simulink library "ovenLib"  (R2016a)
settings: Solver=ode45  StartTime=0.0  StopTime=10.0  RelTol=1e-3
undefined symbols (not defined in the file): des, N
libraries: fl_lib x33, simulink x18, nesl_utility x11, PJPhysLib_lib x3
(part 1 of 2)
settings Model: Creator=peter  LastModifiedBy=peter
settings DataIOCC: LimitDataPoints=on  SaveFormat=Array
settings HardwareCC: ProdBitPerPointer=32  ProdLargestAtomicFloat=None  ProdIntDivRoundTo=Undefined  ProdEndianess=Unspecified  ProdWordSize=32  ProdHWDeviceType=32-bit Generic
settings ModelReferenceCC: PropagateSignalLabelsOutOfModel=off
settings ConfigComp: CovModelRefEnable=Off

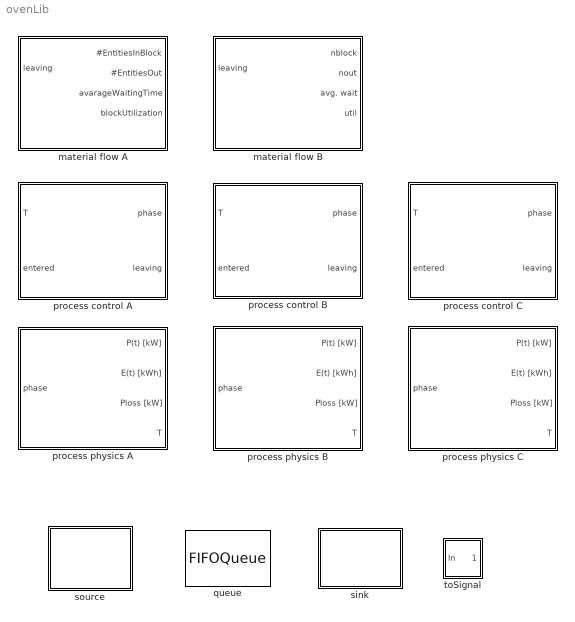
== system ovenLib ==
  material flow A : Subsystem  mask{N=6}
      mask prompts: N "oven capacity"
      mask Display:
      | text(0.1, 0.55, '\fontsize{24} MF (A)', 'texmode', 'on')
      | port_label('input', 1, 'leaving')
      | port_label('output', 2, 'nOut')
      | port_label('output', 1, 'nBlock')
      | port_label('output', 3, 'avg. wait')
      | port_label('output', 4, 'util.')
  material flow B : Subsystem  mask{N=N}
      mask prompts: N "oven capacity"
      mask Display:
      | text(0.1, 0.55, '\fontsize{24} MF (B)', 'texmode', 'on')
      | port_label('input', 1, 'leaving')
      | port_label('output', 2, 'nOut')
      | port_label('output', 1, 'nBlock')
      | port_label('output', 3, 'avg. wait')
      | port_label('output', 4, 'util.')
  process control A : Subsystem  mask{tH=70, Tset=800, N=6}
      mask prompts: tH "heating time [min]"; Tset "heating temperature [°C]"; N "oven capacity"
      mask Display:
      | disp('\fontsize{24} PC (A)', 'texmode', 'on')
      | port_label('input', 1, 'T')
      | port_label('input', 2, 'entered')
      | port_label('output', 1, 'phase')
      | port_label('output', 2, 'leaving')
  process control B : Subsystem  mask{HeatProgram=[40 400; 30 800], N=6}
      mask prompts: HeatProgram "heating program"; N "oven capacity"
      mask Display:
      | disp('\fontsize{24} PC (B)', 'texmode', 'on')
      | port_label('input', 1, 'T')
      | port_label('input', 2, 'entered')
      | port_label('output', 1, 'phase')
      | port_label('output', 2, 'leaving')
  process control C : Subsystem  mask{T0C=0, Tcool=30, N=6, HeatProgram=[0 20; 30 400;70 400;110 800;140 800]}
      mask prompts: T0C "0 °C in K"; Tcool "cooling temperature [°C]"; N "oven capacity"; HeatProgram "heating program"
      mask init:
      | T0C = 273.15;
      mask Display:
      | disp('\fontsize{24} PC (C)', 'texmode', 'on')
      | port_label('input', 1, 'T')
      | port_label('input', 2, 'entered')
      | port_label('output', 1, 'phase')
      | port_label('output', 2, 'leaving')
  process physics A : Subsystem  mask{Te=20, T_o=20, m_o=70, PH=8000, cp_o=1000, k_A=6.4, P0=2000}
      mask prompts: Te "environment temperature [°C]"; T_o "initial oven temperature [°C]"; m_o "oven mass [kg]"; PH "heating power [W]"; cp_o "oven specific heat capacity [J/(kg*K)]"; k_A "heat transfer coefficient * area [W/K]"; P0 "basic oven load [W]"
      mask init:
      | T0C = 273.15;
      | sigma = 5.67e-8;
      mask Display:
      | text(0.2, 0.55, '\fontsize{24} PP (A)', 'texmode', 'on')
      | port_label('input', 1, 'phase')
      | port_label('output', 1, 'P(t)')
      | port_label('output', 2, 'E(t)')
      | port_label('output', 3, 'Ploss(t)')
      | port_label('output', 4, 'T')
  process physics B : Subsystem  mask{T0C=0, sigma=0, Tu=20, T_o=20, m_o=70, PH=8000, cp_o=1000, etaO=0.95, alpha=28, epsilon=0.22, k_A=6.4, A_t=0.2, Pgrund=2000, m_w=1.4, cp_w=480, A_w_k=0.02, A_w_s=0.02, T_w=20}
      mask prompts: T0C "0°C in K"; sigma "Stefan Boltzmann constant"; Tu "environment temperature [°C]"; T_o "initial oven temperature [°C]"; m_o "oven mass [kg]"; PH "heating power [W]"; cp_o "oven specific heat capacity [J/(kg*K)]"; etaO "oven efficiency"; alpha "heat transfer coefficient [W/(m^2*K)]"; epsilon "emissivity"; k_A "heat transfer coefficient * area [W/K]"; A_t "area of oven door [m^2]"; Pgrund "basic oven load [W]"; m_w "work piece mass [kg]"; cp_w "work piece specific heat capacity [J/(kg*K)]"; A_w_k "work piece convective area [m^2]"; A_w_s "work piece radiation area [m^2]"; T_w "initial work piece temperature [°C]"
      mask init:
      | T0C = 273.15;
      | sigma = 5.67e-8;
      mask Display:
      | text(0.2, 0.55, '\fontsize{24} PP (B)', 'texmode', 'on')
      | port_label('input', 1, 'phase')
      | port_label('output', 1, 'P(t)')
      | port_label('output', 2, 'E(t)')
      | port_label('output', 3, 'Ploss(t)')
      | port_label('output', 4, 'T')
  process physics C : Subsystem  mask{T0C=0, sigma=0, Tu=20, T_o=20, m_o=70, PH=8000, cp_o=1000, etaO=0.95, alpha=28, epsilon=0.22, k_A=6.4, A_t=0.2, Pgrund=2000, m_w=1.4, cp_w=480, A_w_k=0.02, A_w_s=0.02, T_w=20}
      mask prompts: T0C "0°C in K"; sigma "Stefan Boltzmann constant"; Tu "environment temperature [°C]"; T_o "initial oven temperature [°C]"; m_o "oven mass [kg]"; PH "heating power [W]"; cp_o "oven specific heat capacity [J/(kg*K)]"; etaO "oven efficiency"; alpha "heat transfer coefficient [W/(m^2*K)]"; epsilon "emissivity"; k_A "heat transfer coefficient * area [W/K]"; A_t "area of oven door [m^2]"; Pgrund "basic oven load [W]"; m_w "work piece mass [kg]"; cp_w "work piece specific heat capacity [J/(kg*K)]"; A_w_k "work piece convective area [m^2]"; A_w_s "work piece radiation area [m^2]"; T_w "initial work piece temperature [°C]"
      mask init:
      | T0C = 273.15;
      | sigma = 5.67e-8;
      mask Display:
      | text(0.2, 0.55, '\fontsize{24} PP (C)', 'texmode', 'on')
      | port_label('input', 1, 'phase')
      | port_label('output', 1, 'P(t)')
      | port_label('output', 2, 'E(t)')
      | port_label('output', 3, 'Ploss(t)')
      | port_label('output', 4, 'T')
  queue : FIFOQueue  Capacity=inf
  sink : Subsystem  mask{nParts=25}
      mask prompts: nParts "Anzahl der bearbeiteten Werkstuecke"
  source : Subsystem  mask{nParts=25, period=0.1, parts=|, htz=100Cr6}
      mask parts=|
      | [-110 -110    0    0 -110    0    0    0    0    0    0    0    0    0    0    0    0    0    0    0
      |    0   60   60    0    0    0    0    0    0    0    0    0    0    0    0    0    0    0    0    0
      |    0    0    0    0    0    0    0    0    0    0    0    0    0    0    0    0    0    0    0    0
      |    0    0    0    0    0    0    0    0    0    0    0    0    0    0    0    0    0    0    0    0
      | ]
      mask prompts: nParts "Anzahl der zu generierende Werkstuecke"; period "Transferzeit in [s]"; parts "Rohteilgeometrie"; htz "Werkstoff"
      mask TypeOptions htz: 100Cr6 | 42CrMo4
  toSignal : Subsystem

== system ovenLib/material flow A ==
  leaving : Inport
  N-Server : NServer  NumberOfServers=N  ServiceTime=0  StatNumberDeparted=on  StatNumberInBlock=on  StatAverageWait=on  StatUtilization=on
      settings: OutputPortMap=o0,o1,o4,o5
  Release Gate : ReleaseGate  OpenGateUpon=Function call from port fcn
  IN : PMIOPort  Port=1  Side=Left
  OUT : PMIOPort  Port=2  Side=Right
  #EntitiesInBlock : Outport
  #EntitiesOut : Outport  Port=2
  avarageWaitingTime : Outport  Port=3
  blockUtilization : Outport  Port=4
  wires:
  leaving/1 -> Release Gate/1
  N-Server/3 -> avarageWaitingTime/1
  N-Server/1 -> #EntitiesOut/1
  N-Server/2 -> #EntitiesInBlock/1
  N-Server/4 -> blockUtilization/1
  connections:
  IN/RConn1 -- N-Server/LConn1
  N-Server/RConn1 -- Release Gate/LConn1
  Release Gate/RConn1 -- OUT/RConn1

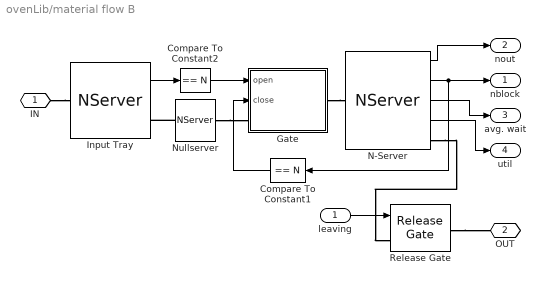
== system ovenLib/material flow B ==
  leaving : Inport
  Compare To Constant1 : simulink/Logic and Bit Operations/Compare To Constant  relop===  const=N  OutDataTypeStr=boolean
  Compare To Constant2 : simulink/Logic and Bit Operations/Compare To Constant  relop===  const=N  OutDataTypeStr=boolean
  Gate : Subsystem  mask(Gate){}
      mask help:
      | Gate for Entities that can be opened or closed via rising trigger inputs.
      | It is  initially open.
  Input Tray : NServer  NumberOfServers=N  ServiceTime=0  StatNumberInBlock=on
      settings: OutputPortMap=o1
  N-Server : NServer  NumberOfServers=N  ServiceTime=0  StatNumberDeparted=on  StatNumberInBlock=on  StatAverageWait=on  StatUtilization=on
      settings: OutputPortMap=o0,o1,o4,o5
  Nullserver : NServer  NumberOfServers=1  ServiceTime=0
  Release Gate : ReleaseGate  OpenGateUpon=Function call from port fcn
  IN : PMIOPort  Port=1  Side=Left
  OUT : PMIOPort  Port=2  Side=Right
  nblock : Outport
  nout : Outport  Port=2
  avg. wait : Outport  Port=3
  util : Outport  Port=4
  wires:
  Input Tray/1 -> Compare To Constant2/1
  Compare To Constant2/1 -> Gate/1(open)
  leaving/1 -> Release Gate/1
  Compare To Constant1/1 -> Gate/2(close)
  N-Server/1 -> nout/1
  N-Server/3 -> avg. wait/1
  N-Server/2 -> Compare To Constant1/1, nblock/1
  N-Server/4 -> util/1
  connections:
  Nullserver/RConn1 -- Gate/LConn1
  Nullserver/LConn1 -- Input Tray/RConn1
  Release Gate/RConn1 -- OUT/RConn1
  Gate/RConn1 -- N-Server/LConn1
  IN/RConn1 -- Input Tray/LConn1
  N-Server/RConn1 -- Release Gate/LConn1

== system ovenLib/process control A ==
  T : Inport
  entered : Inport  Port=2
  Constant1 : Constant  Value=0
  Event to Timed Signal1 : EventToTimedSignal
  MinMax : MinMax  Function=max  Inputs=5
  create control entity : Subsystem
  destroy control entity : Subsystem
  gate control : Subsystem  TreatAsAtomicUnit=on
  phase 1 load : Subsystem  mask{ts=5}
      mask prompts: ts "Service Time [min]"
  phase 2 heatUp : Subsystem
  phase 3 hold : Subsystem
  phase 4 unload : Subsystem  mask{ts=5}
      mask prompts: ts "Service Time [min]"
  phase : Outport
  leaving : Outport  Port=2
  wires:
  T/1 -> phase 2 heatUp/1(T)
  phase 1 load/1(Phase) -> MinMax/2
  phase 2 heatUp/1(Phase) -> MinMax/3
  phase 3 hold/1(Phase) -> MinMax/4
  Constant1/1 -> MinMax/1
  MinMax/1 -> Event to Timed Signal1/1
  phase 4 unload/1(Phase) -> MinMax/5
  gate control/1(fN) -> leaving/1
  Event to Timed Signal1/1 -> phase/1
  entered/1 -> create control entity/1(#n)
  destroy control entity/1(trigger) -> gate control/Trigger
  connections:
  phase 3 hold/LConn1 -- phase 2 heatUp/RConn1
  phase 3 hold/RConn1 -- phase 4 unload/LConn1
  phase 1 load/RConn1 -- phase 2 heatUp/LConn1
  create control entity/RConn1 -- phase 1 load/LConn1
  destroy control entity/LConn1 -- phase 4 unload/RConn1

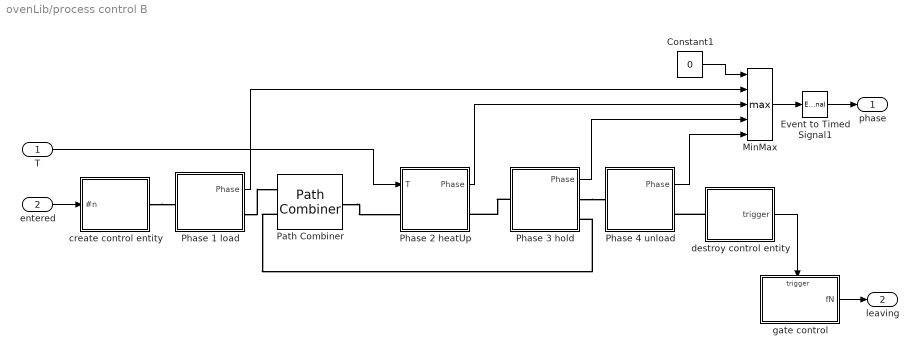
== system ovenLib/process control B ==
  T : Inport
  entered : Inport  Port=2
  Constant1 : Constant  Value=0
  Event to Timed Signal1 : EventToTimedSignal
  MinMax : MinMax  Function=max  Inputs=5
  Path Combiner : PathCombiner  NumberInputPorts=2
  Phase 1 load : Subsystem  mask{ts=5}
      mask prompts: ts "Service Time [min]"
  Phase 2 heatUp : Subsystem
  Phase 3 hold : Subsystem
  Phase 4 unload : Subsystem  mask{ts=5}
      mask prompts: ts "Service Time [min]"
  create control entity : Subsystem
  destroy control entity : Subsystem
  gate control : Subsystem  TreatAsAtomicUnit=on
  phase : Outport
  leaving : Outport  Port=2
  wires:
  destroy control entity/1(trigger) -> gate control/Trigger
  entered/1 -> create control entity/1(#n)
  Event to Timed Signal1/1 -> phase/1
  gate control/1(fN) -> leaving/1
  T/1 -> Phase 2 heatUp/1(T)
  Phase 4 unload/1(Phase) -> MinMax/5
  MinMax/1 -> Event to Timed Signal1/1
  Constant1/1 -> MinMax/1
  Phase 3 hold/1(Phase) -> MinMax/4
  Phase 2 heatUp/1(Phase) -> MinMax/3
  Phase 1 load/1(Phase) -> MinMax/2
  connections:
  destroy control entity/LConn1 -- Phase 4 unload/RConn1
  create control entity/RConn1 -- Phase 1 load/LConn1
  Path Combiner/RConn1 -- Phase 2 heatUp/LConn1
  Path Combiner/LConn2 -- Phase 3 hold/RConn2
  Phase 3 hold/RConn1 -- Phase 4 unload/LConn1
  Phase 1 load/RConn1 -- Path Combiner/LConn1
  Phase 3 hold/LConn1 -- Phase 2 heatUp/RConn1

== system ovenLib/process control C ==
  T : Inport
  entered : Inport  Port=2
  Constant16 : Constant  Value=N
  Constant17 : Constant  Value=HeatProgram
  DEVS : Stateflow chart  TreatAsAtomicUnit=on
  Event to Timed Signal1 : EventToTimedSignal
  Event to Timed Signal2 : EventToTimedSignal
  Mux : Mux
  Signal-Based Function-Call Generator : SignalBasedFunctionCallGenerator
      settings: InputPortMap=u1
  checkTemperature : Subsystem
  schedTEvent : Subsystem
  phase : Outport
  leaving : Outport  Port=2
  wires:
  entered/1 -> Signal-Based Function-Call Generator/1
  Event to Timed Signal2/1 -> phase/1, checkTemperature/1(phase)
  Event to Timed Signal1/1 -> checkTemperature/2(Tset)
  checkTemperature/2(coolDownReady) -> Mux/4
  checkTemperature/1(heatUpReady) -> Mux/3
  schedTEvent/1(wakeUp) -> Mux/2
  Signal-Based Function-Call Generator/1 -> Mux/1
  DEVS/2(Tset) -> Event to Timed Signal1/1
  Constant17/1 -> DEVS/2(HeatP)
  Constant16/1 -> DEVS/1(max_capa)
  DEVS/3(phase) -> Event to Timed Signal2/1
  DEVS/4(newSigma()) -> schedTEvent/1(newSigma)
  DEVS/1(sigma) -> schedTEvent/2(sigma)
  DEVS/5(openGate()) -> leaving/1
  Mux/1 -> DEVS/Trigger
  T/1 -> checkTemperature/3(T)

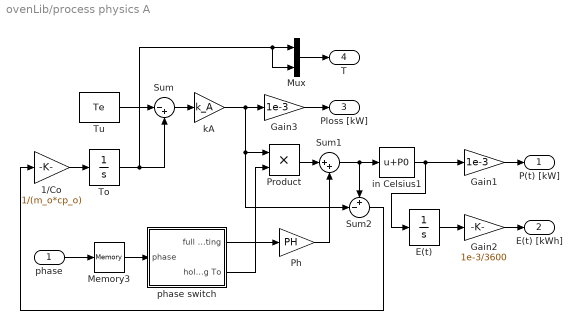
== system ovenLib/process physics A ==
  phase : Inport
  1/Co : Gain  Gain=1/(m_o*cp_o)
  E(t) : Integrator
  Gain1 : Gain  Gain=1e-3
  Gain2 : Gain  Gain=1e-3/3600
  Gain3 : Gain  Gain=1e-3
  Memory3 : Memory  InheritSampleTime=on
  Mux : Mux  Inputs=2
  Ph : Gain  Gain=PH
  Product : Product
  Sum : Sum  Inputs=|-+
  Sum1 : Sum  Inputs=|++
  Sum2 : Sum  Inputs=+-|
  To : Integrator  InitialCondition=T_o
  Tu : Constant  Value=Te
  in Celsius1 : Bias  Bias=P0
  kA : Gain  Gain=k_A
  phase switch : Subsystem
  P(t) [kW] : Outport
  E(t) [kWh] : Outport  Port=2
  Ploss [kW] : Outport  Port=3
  T : Outport  Port=4
  wires:
  Gain2/1 -> E(t) [kWh]/1
  E(t)/1 -> Gain2/1
  in Celsius1/1 -> E(t)/1, Gain1/1
  Sum/1 -> kA/1
  Gain3/1 -> Ploss [kW]/1
  Gain1/1 -> P(t) [kW]/1
  Memory3/1 -> phase switch/1(phase)
  phase/1 -> Memory3/1
  Sum2/1 -> 1/Co/1
  1/Co/1 -> To/1
  Sum1/1 -> in Celsius1/1, Sum2/1
  Product/1 -> Sum1/1
  Ph/1 -> Sum1/2
  phase switch/1(full heating) -> Ph/1
  phase switch/2(holding To) -> Product/2
  kA/1 -> Sum2/2, Product/1, Gain3/1
  Tu/1 -> Sum/1
  To/1 -> Sum/2, Mux/1, Mux/2
  Mux/1 -> T/1

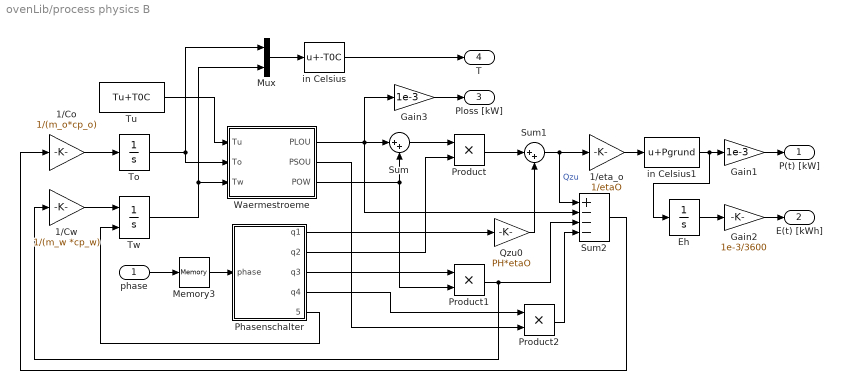
== system ovenLib/process physics B ==
  phase : Inport
  1/Co : Gain  Gain=1/(m_o*cp_o)
  1/Cw : Gain  Gain=1/(m_w *cp_w)
  1/eta_o : Gain  Gain=1/etaO
  Eh : Integrator
  Gain1 : Gain  Gain=1e-3
  Gain2 : Gain  Gain=1e-3/3600
  Gain3 : Gain  Gain=1e-3
  Memory3 : Memory  InheritSampleTime=on
  Mux : Mux  Inputs=2
  Phasenschalter : Subsystem
  Product : Product
  Product1 : Product
  Product2 : Product
  Qzu0 : Gain  Gain=PH*etaO
  Sum : Sum  Inputs=|++
  Sum1 : Sum  Inputs=|++
  Sum2 : Sum  Inputs=+---
  To : Integrator  InitialCondition=T_w + T0C
  Tu : Constant  Value=Tu+T0C
  Tw : Integrator  ExternalReset=rising  InitialCondition=T_w + T0C
  Waermestroeme : Subsystem
  in Celsius : Bias  Bias=-T0C
  in Celsius1 : Bias  Bias=Pgrund
  P(t) [kW] : Outport
  E(t) [kWh] : Outport  Port=2
  Ploss [kW] : Outport  Port=3
  T : Outport  Port=4
  wires:
  Gain2/1 -> E(t) [kWh]/1
  Eh/1 -> Gain2/1
  Gain3/1 -> Ploss [kW]/1
  Gain1/1 -> P(t) [kW]/1
  Memory3/1 -> Phasenschalter/1(phase)
  phase/1 -> Memory3/1
  To/1 -> Mux/1, Waermestroeme/2(To)
  Phasenschalter/5(restartTw) -> Tw/2
  Phasenschalter/4(q4) -> Product2/1
  in Celsius1/1 -> Gain1/1, Eh/1
  1/eta_o/1 -> in Celsius1/1
  Sum2/1 -> 1/Co/1
  Product2/1 -> Sum2/4
  Waermestroeme/2(PSOU) -> Product2/2
  Product1/1 -> Sum2/3, 1/Cw/1
  Phasenschalter/3(q3) -> Product1/1
  1/Cw/1 -> Tw/1
  1/Co/1 -> To/1
  Sum1/1 -> Sum2/1, 1/eta_o/1  "Qzu"
  Product/1 -> Sum1/1
  Qzu0/1 -> Sum1/2
  Phasenschalter/1(q1) -> Qzu0/1
  Phasenschalter/2(q2) -> Product/2
  Sum/1 -> Product/1
  Waermestroeme/3(POW) -> Sum/2, Product1/2
  Waermestroeme/1(PLOU) -> Gain3/1, Sum2/2, Sum/1
  Tu/1 -> Waermestroeme/1(Tu)
  in Celsius/1 -> T/1
  Mux/1 -> in Celsius/1
  Tw/1 -> Waermestroeme/3(Tw), Mux/2

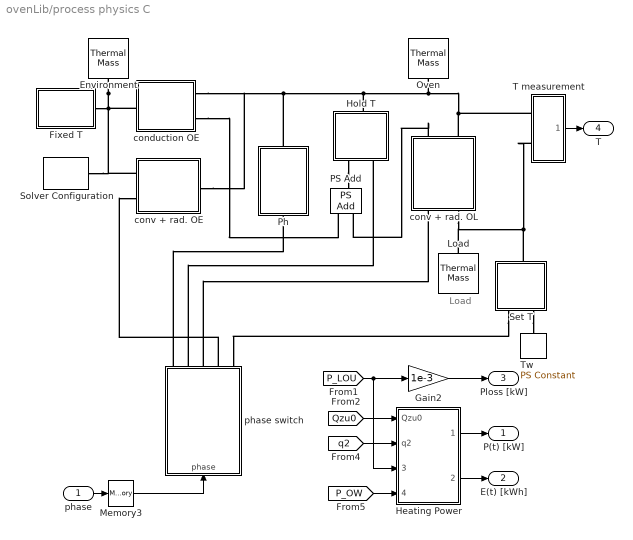
== system ovenLib/process physics C ==
  note: Load
  phase : Inport
  Environment : fl_lib/Thermal/Thermal Elements/Thermal Mass  mass=1000 kg  sp_heat=2000 J/kg/K  T_specify=on  T_priority=High  T=360 K  Q_specify=off  Q_priority=High  Q=0 J/s
  Fixed T : Subsystem
  Gain2 : Gain  Gain=1e-3
  Heating Power : Subsystem
  Hold T : Subsystem
  Load : fl_lib/Thermal/Thermal Elements/Thermal Mass  mass=m_w kg  sp_heat=cp_w J/kg/K  T_specify=on  T_priority=High  T=T_w K  Q_specify=off  Q_priority=High  Q=0 J/s
  Memory3 : Memory  InheritSampleTime=on
  Oven : fl_lib/Thermal/Thermal Elements/Thermal Mass  mass=m_o kg  sp_heat=cp_o J/kg/K  T_specify=on  T_priority=High  T=T_o K  Q_specify=off  Q_priority=High  Q=0 J/s
  PS Add : fl_lib/Physical Signals/Functions/PS Add
  Ph : Subsystem
  Set T : Subsystem
  Solver Configuration : nesl_utility/Solver Configuration  PhysicalDomain=network_engine_domain  SubClassName=solver  LeftPortType=input  RightPortType=generic  Accelerate=off  Tones=[]  Harmonics=[]  SimulateNoise=off  Profile=off  UseLocalSampling=off  EnableSwitchedLinearOptims=on  FrequencyDomain=off  UseCCode=off  RelTol=0.001  AbsTol=1e-06  MinStep=1e-09  ToWorkspace=off  RevertToSquareIcSolve=off  NumHomotopyIterations=100  PhasorMode=off  PhasorModeNumHarmonics=1  OverrideAbsTol=off  DoDC=off  ResidualTolerance=1e-09  UseLocalSolver=off  LocalSolverChoice=NE_BACKWARD_EULER_ADVANCER  LocalSolverSampleTime=0.001  DoFixedCost=off  MaxNonlinIter=3  MaxModeIter=2  LinearAlgebra=Sparse  DelaysMemoryBudget=1024  AutomaticFiltering=on  FilteringTimeConstant=0.001
  T measurement : Subsystem
      mask Display: image('thermometer.png')
  Tw : fl_lib/Physical Signals/Sources/PS Constant  constant=T_w + T0C
  conduction OE : Subsystem
  conv + rad. OL : Subsystem
  conv + rad. OE : Subsystem
  phase switch : Subsystem
  P(t) [kW] : Outport
  E(t) [kWh] : Outport  Port=2
  Ploss [kW] : Outport  Port=3
  T : Outport  Port=4
  wires:
  Heating Power/2(E(t) [kWh]) -> E(t) [kWh]/1
  Gain2/1 -> Ploss [kW]/1
  Heating Power/1(P(t) [kW]) -> P(t) [kW]/1
  [Qzu0] -> Heating Power/1(Qzu0)
  [q2] -> Heating Power/2(q2)
  [P_LOU] -> Heating Power/3(P_LOU), Gain2/1
  [P_OW] -> Heating Power/4(P_OW)
  phase/1 -> Memory3/1
  Memory3/1 -> phase switch/1(phase)
  T measurement/1(Out1) -> T/1
  connections:
  Environment/LConn1 -- conv + rad. OE/LConn1 -- Solver Configuration/RConn1 -- conduction OE/LConn1 -- Fixed T/RConn1
  Ph/RConn1 -- conv + rad. OE/RConn1 -- conduction OE/RConn1 -- Oven/LConn1 -- T measurement/LConn1 -- conv + rad. OL/RConn2 -- Hold T/RConn1
  Set T/RConn1 -- T measurement/LConn2 -- Load/LConn1 -- conv + rad. OL/LConn2
  Set T/LConn1 -- phase switch/RConn5
  Set T/LConn2 -- Tw/RConn1
  conduction OE/RConn2 -- PS Add/LConn2
  conv + rad. OL/RConn1 -- PS Add/LConn1
  phase switch/RConn1 -- Ph/LConn1
  Hold T/LConn1 -- PS Add/RConn1
  phase switch/RConn4 -- conv + rad. OE/LConn2
  phase switch/RConn3 -- conv + rad. OL/LConn1
  phase switch/RConn2 -- Hold T/LConn2

== system ovenLib/sink ==
  Constant : Constant  Value=nParts
  Entity Sink : EntitySink  StatNumberArrived=on
  Event to Timed Signal : EventToTimedSignal
  Relational Operator : RelationalOperator  Operator===  OutDataTypeStr=boolean
  Stop Simulation : Stop
  IN : PMIOPort  Port=1  Side=Left
  wires:
  Relational Operator/1 -> Event to Timed Signal/1
  Event to Timed Signal/1 -> Stop Simulation/1
  Constant/1 -> Relational Operator/1
  Entity Sink/1 -> Relational Operator/2
  connections:
  IN/RConn1 -- Entity Sink/LConn1

== system ovenLib/source ==
  Attribute Function : Subsystem  LoadFcn=des.afb.attributefunction_support(gcb,'LoadFcn');  StartFcn=des.afb.attributefunction_support(gcb,'StartFcn');  mask(Attribute Function){OutputNamePrefix=out_}
      mask prompts: OutputNamePrefix "Prefix name"
      settings: CopyFcn=des.afb.attributefunction_support(gcb,'CopyFcn');  OpenFcn=des.afb.attributefunction_support(gcb,'OpenFcn');  ErrorFcn=des.afb.error_redirect
      mask Help: slhelp(gcbh)
      mask Display: image(des_iconLoad('attribFunction.jpg'),'center');
  Constant : Constant  Value=nParts
  Constant1 : Constant  Value=htz
  Constant2 : Constant  Value=parts
  Entity Departure Counter : EntityDepartureCounter  NumberDepartedAttributeName=part_no
  Entity Sink : EntitySink  AvailableForArrivals=off
  Output Switch : OutputSwitch  NumberOutputPorts=2  SwitchingCriterion=From attribute  AttributeName=port
  Set Attribute : SetAttribute  AttributeName=nr_wp  AttributeFrom=Signal port  EvaluatedAttributeValue={ []}
  Set Attribute1 : SetAttribute  AttributeName=htz|parts  AttributeFrom=Signal port|Signal port  AttributeValue=1|1  AttributeTreatAsVector=1|1  EvaluatedAttributeValue={ [];[]}
      settings: InputPortMap=u0,u1
  Single Server1 : SingleServer  ServiceTime=0
  Time-Based Entity Generator : TimeBasedEntityGenerator  Period=period
  OUT : PMIOPort  Port=1  Side=Right
  wires:
  Constant2/1 -> Set Attribute1/2
  Constant1/1 -> Set Attribute1/1
  Constant/1 -> Set Attribute/1
  connections:
  Time-Based Entity Generator/RConn1 -- Entity Departure Counter/LConn1
  Entity Departure Counter/RConn1 -- Set Attribute/LConn1
  Attribute Function/RConn1 -- Single Server1/LConn1
  Set Attribute/RConn1 -- Attribute Function/LConn1
  Output Switch/RConn1 -- Set Attribute1/LConn1
  Output Switch/RConn2 -- Entity Sink/LConn1
  Set Attribute1/RConn1 -- OUT/RConn1
  Single Server1/RConn1 -- Output Switch/LConn1

== system ovenLib/toSignal ==
  In : Inport
  toSIgnal : EventToTimedSignal
  Out : Outport
  wires:
  toSIgnal/1 -> Out/1
  In/1 -> toSIgnal/1

== system ovenLib/material flow B/Gate ==
  open : Inport
  close : Inport  Port=2
  Constant : Constant  Value=0
  Constant1 : Constant
  Enabled Gate1 : EnabledGate
  Signal Latch : SignalLatch  WriteMemoryUpon=Trigger from port wtr  ReadMemoryUpon=Trigger from port rtr  MemoryReadEdgeOption=Rising  ReportMemoryState=on  ReportMemoryUponRead=off
      settings: InputPortMap=u0,u1,u2
  Sum : Sum  Inputs=+-|
  IN : PMIOPort  Port=1  Side=Left
  OUT : PMIOPort  Port=2  Side=Right
  wires:
  Sum/1 -> Enabled Gate1/1
  Constant1/1 -> Sum/1
  Signal Latch/1 -> Sum/2
  open/1 -> Signal Latch/2
  close/1 -> Signal Latch/1
  Constant/1 -> Signal Latch/3
  connections:
  Enabled Gate1/LConn1 -- IN/RConn1
  OUT/RConn1 -- Enabled Gate1/RConn1

== system ovenLib/process control A/create control entity ==
  #n : Inport
  Compare To Constant : simulink/Logic and Bit Operations/Compare To Constant  relop===  const=N  OutDataTypeStr=boolean
  Event-Based Entity Generator : EventBasedEntityGenerator
  OUT : PMIOPort  Port=1  Side=Right
  wires:
  #n/1 -> Compare To Constant/1
  Compare To Constant/1 -> Event-Based Entity Generator/1
  connections:
  Event-Based Entity Generator/RConn1 -- OUT/RConn1

== system ovenLib/process control A/destroy control entity ==
  Entity Sink : EntitySink  StatNumberArrived=on
  Signal-Based Function-Call Generator : SignalBasedFunctionCallGenerator
      settings: InputPortMap=u1
  IN : PMIOPort  Port=1  Side=Left
  trigger : Outport
  wires:
  Signal-Based Function-Call Generator/1 -> trigger/1
  Entity Sink/1 -> Signal-Based Function-Call Generator/1
  connections:
  Entity Sink/LConn1 -- IN/RConn1

== system ovenLib/process control A/gate control ==
  Trigger : TriggerPort  TriggerType=function-call  VariantControl=Variant
  Function-Call Generator : simulink/Ports & Subsystems/Function-Call Generator  sample_time=-1  numberOfIterations=N
  fN : Outport
  wires:
  Function-Call Generator/1 -> fN/1

== system ovenLib/process control A/phase 1 load ==
  Server load : SingleServer  ServiceTime=60*ts  StatNumberInBlock=on
      settings: OutputPortMap=o1
  phase : Gain
  OUT : PMIOPort  Port=1  Side=Right
  IN : PMIOPort  Port=2  Side=Left
  Phase : Outport
  wires:
  Server load/1 -> phase/1
  phase/1 -> Phase/1
  connections:
  IN/RConn1 -- Server load/LConn1
  Server load/RConn1 -- OUT/RConn1

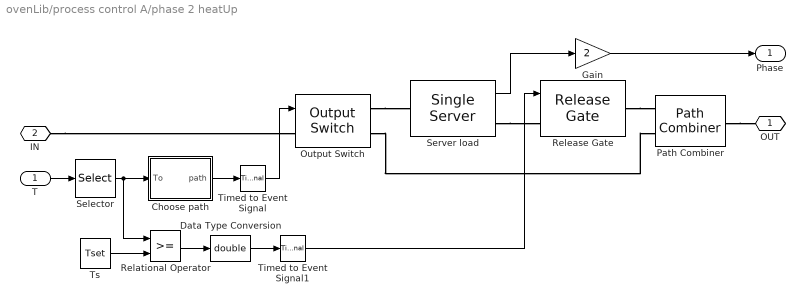
== system ovenLib/process control A/phase 2 heatUp ==
  T : Inport
  Choose path : Subsystem
  Data Type Conversion : DataTypeConversion  OutDataTypeStr=double
  Gain : Gain  Gain=2
  Output Switch : OutputSwitch  NumberOutputPorts=2  SwitchingCriterion=From signal port p  InitialConditionsOpt=on
  Path Combiner : PathCombiner  NumberInputPorts=2
  Relational Operator : RelationalOperator  OutDataTypeStr=boolean
  Release Gate : ReleaseGate
  Selector : Selector  InputPortWidth=2  IndexOptions=Index vector (dialog)  Indices=[1]  OutputSizes=1
  Server load : SingleServer  ServiceTime=0  StatNumberInBlock=on
      settings: OutputPortMap=o1
  Timed to Event Signal : TimedToEventSignal
  Timed to Event Signal1 : TimedToEventSignal
  Ts : Constant  Value=Tset
  OUT : PMIOPort  Port=1  Side=Right
  IN : PMIOPort  Port=2  Side=Left
  Phase : Outport
  wires:
  Timed to Event Signal/1 -> Output Switch/1
  Timed to Event Signal1/1 -> Release Gate/1
  Data Type Conversion/1 -> Timed to Event Signal1/1
  Relational Operator/1 -> Data Type Conversion/1
  Ts/1 -> Relational Operator/2
  Server load/1 -> Gain/1
  Gain/1 -> Phase/1
  T/1 -> Selector/1
  Choose path/1(path) -> Timed to Event Signal/1
  Selector/1 -> Choose path/1(To), Relational Operator/1
  connections:
  Server load/RConn1 -- Release Gate/LConn1
  IN/RConn1 -- Output Switch/LConn1
  Output Switch/RConn1 -- Server load/LConn1
  Release Gate/RConn1 -- Path Combiner/LConn1
  Path Combiner/RConn1 -- OUT/RConn1
  Output Switch/RConn2 -- Path Combiner/LConn2

== system ovenLib/process control A/phase 3 hold ==
  Gain : Gain  Gain=3
  Server load : SingleServer  ServiceTime=tH*60  StatNumberInBlock=on
      settings: OutputPortMap=o1
  IN : PMIOPort  Port=1  Side=Left
  OUT1 : PMIOPort  Port=2  Side=Right
  Phase : Outport
  wires:
  Gain/1 -> Phase/1
  Server load/1 -> Gain/1
  connections:
  Server load/LConn1 -- IN/RConn1
  Server load/RConn1 -- OUT1/RConn1

== system ovenLib/process control A/phase 4 unload ==
  Gain : Gain  Gain=4
  Server load : SingleServer  ServiceTime=60*ts  StatNumberInBlock=on
      settings: OutputPortMap=o1
  OUT : PMIOPort  Port=1  Side=Right
  IN : PMIOPort  Port=2  Side=Left
  Phase : Outport
  wires:
  Server load/1 -> Gain/1
  Gain/1 -> Phase/1
  connections:
  Server load/RConn1 -- OUT/RConn1
  IN/RConn1 -- Server load/LConn1

== system ovenLib/process control B/Phase 1 load ==
  Server load : SingleServer  ServiceTime=60*ts  StatNumberInBlock=on
      settings: OutputPortMap=o1
  Set HeatP number : SetAttribute  AttributeName=nextHeatPNo|HeatP  AttributeFrom=Dialog|Dialog  AttributeValue=1|HeatProgram  AttributeTreatAsVector=1|1  EvaluatedAttributeValue={ 1;HeatProgram}
  phase : Gain
  OUT : PMIOPort  Port=1  Side=Right
  IN : PMIOPort  Port=2  Side=Left
  Phase : Outport
  wires:
  phase/1 -> Phase/1
  Server load/1 -> phase/1
  connections:
  Set HeatP number/RConn1 -- OUT/RConn1
  IN/RConn1 -- Server load/LConn1
  Server load/RConn1 -- Set HeatP number/LConn1

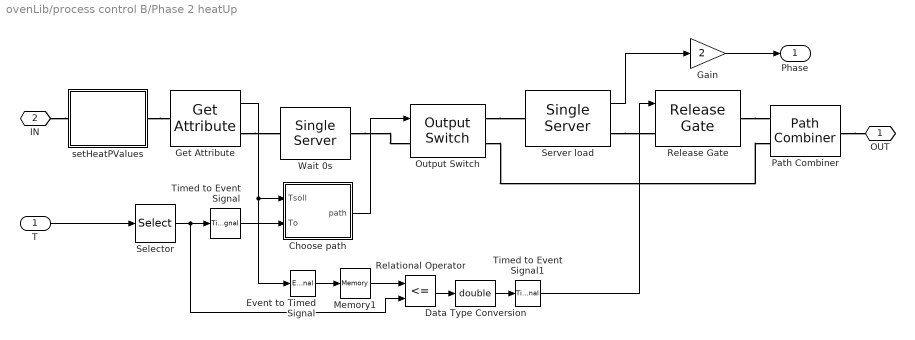
== system ovenLib/process control B/Phase 2 heatUp ==
  T : Inport
  Choose path : Subsystem  TreatAsAtomicUnit=on
  Data Type Conversion : DataTypeConversion  OutDataTypeStr=double
  Event to Timed Signal : EventToTimedSignal
  Gain : Gain  Gain=2
  Get Attribute : GetAttribute  AttributeName=HeatPTemp  EvaluatedDefaultAttributeValue={ []}
      settings: OutputPortMap=o1
  Memory1 : Memory
  Output Switch : OutputSwitch  NumberOutputPorts=2  SwitchingCriterion=From signal port p  InitialConditionsOpt=on
  Path Combiner : PathCombiner  NumberInputPorts=2
  Relational Operator : RelationalOperator  Operator=<=  OutDataTypeStr=boolean
  Release Gate : ReleaseGate
  Selector : Selector  InputPortWidth=2  IndexOptions=Index vector (dialog)  Indices=[1]  OutputSizes=1
  Server load : SingleServer  ServiceTime=0  StatNumberInBlock=on
      settings: OutputPortMap=o1
  Timed to Event Signal : TimedToEventSignal
  Timed to Event Signal1 : TimedToEventSignal
  Wait 0s : SingleServer  ServiceTime=0
  setHeatPValues : Subsystem  LoadFcn=des.afb.attributefunction_support(gcb,'LoadFcn');  StartFcn=des.afb.attributefunction_support(gcb,'StartFcn');  mask(Attribute Function){OutputNamePrefix=out_}
      mask prompts: OutputNamePrefix "Prefix name"
      settings: CopyFcn=des.afb.attributefunction_support(gcb,'CopyFcn');  OpenFcn=des.afb.attributefunction_support(gcb,'OpenFcn');  ErrorFcn=des.afb.error_redirect
      mask Help: slhelp(gcbh)
      mask Display: image(des_iconLoad('attribFunction.jpg'),'center');
  OUT : PMIOPort  Port=1  Side=Right
  IN : PMIOPort  Port=2  Side=Left
  Phase : Outport
  wires:
  Timed to Event Signal/1 -> Choose path/2(To)
  Timed to Event Signal1/1 -> Release Gate/1
  Data Type Conversion/1 -> Timed to Event Signal1/1
  Relational Operator/1 -> Data Type Conversion/1
  Event to Timed Signal/1 -> Memory1/1
  Memory1/1 -> Relational Operator/1
  T/1 -> Selector/1
  Selector/1 -> Relational Operator/2, Timed to Event Signal/1
  Choose path/1(path) -> Output Switch/1
  Get Attribute/1 -> Choose path/1(Tsoll), Event to Timed Signal/1
  Gain/1 -> Phase/1
  Server load/1 -> Gain/1
  connections:
  Get Attribute/RConn1 -- Wait 0s/LConn1
  Output Switch/RConn2 -- Path Combiner/LConn2
  Path Combiner/RConn1 -- OUT/RConn1
  Release Gate/RConn1 -- Path Combiner/LConn1
  Output Switch/RConn1 -- Server load/LConn1
  Wait 0s/RConn1 -- Output Switch/LConn1
  setHeatPValues/RConn1 -- Get Attribute/LConn1
  IN/RConn1 -- setHeatPValues/LConn1
  Server load/RConn1 -- Release Gate/LConn1

== system ovenLib/process control B/Phase 3 hold ==
  Gain : Gain  Gain=3
  Get Attribute : GetAttribute  AttributeName=HeatPTime  EvaluatedDefaultAttributeValue={ []}
      settings: OutputPortMap=o1
  Output Switch : OutputSwitch  NumberOutputPorts=2  SwitchingCriterion=From attribute  AttributeName=OutPort
  Server load : SingleServer  ServiceTimeFrom=Signal port t  ServiceTime=ts  StatNumberInBlock=on
      settings: OutputPortMap=o1
  Set Out Port : Subsystem  LoadFcn=des.afb.attributefunction_support(gcb,'LoadFcn');  StartFcn=des.afb.attributefunction_support(gcb,'StartFcn');  mask(Attribute Function){OutputNamePrefix=out_}
      mask prompts: OutputNamePrefix "Prefix name"
      settings: CopyFcn=des.afb.attributefunction_support(gcb,'CopyFcn');  OpenFcn=des.afb.attributefunction_support(gcb,'OpenFcn');  ErrorFcn=des.afb.error_redirect
      mask Help: slhelp(gcbh)
      mask Display: image(des_iconLoad('attribFunction.jpg'),'center');
  Sum : Sum  Inputs=|+++
  Wait 0s : SingleServer  ServiceTime=0  StatNumberInBlock=on
      settings: OutputPortMap=o1
  "Wait 0s " : SingleServer  ServiceTime=0  StatNumberInBlock=on
      settings: OutputPortMap=o1
  IN : PMIOPort  Port=1  Side=Left
  OUT1 : PMIOPort  Port=2  Side=Right
  OUT2 : PMIOPort  Port=3  Side=Right
  Phase : Outport
  wires:
  "Wait 0s "/1 -> Sum/3
  Server load/1 -> Sum/2
  Wait 0s/1 -> Sum/1
  Sum/1 -> Gain/1
  Get Attribute/1 -> Server load/1
  Gain/1 -> Phase/1
  connections:
  Server load/RConn1 -- Set Out Port/LConn1
  Output Switch/RConn1 -- OUT1/RConn1
  "Wait 0s "/RConn1 -- Output Switch/LConn1
  Output Switch/RConn2 -- OUT2/RConn1
  Set Out Port/RConn1 -- "Wait 0s "/LConn1
  Wait 0s/RConn1 -- Server load/LConn1
  Get Attribute/RConn1 -- Wait 0s/LConn1
  IN/RConn1 -- Get Attribute/LConn1

== system ovenLib/process control B/Phase 4 unload ==
  Gain : Gain  Gain=4
  Server load : SingleServer  ServiceTime=60*ts  StatNumberInBlock=on
      settings: OutputPortMap=o1
  OUT : PMIOPort  Port=1  Side=Right
  IN : PMIOPort  Port=2  Side=Left
  Phase : Outport
  wires:
  Gain/1 -> Phase/1
  Server load/1 -> Gain/1
  connections:
  IN/RConn1 -- Server load/LConn1
  Server load/RConn1 -- OUT/RConn1

== system ovenLib/process control B/create control entity ==
  #n : Inport
  Compare To Constant : simulink/Logic and Bit Operations/Compare To Constant  relop===  const=N  OutDataTypeStr=boolean
  Event-Based Entity Generator : EventBasedEntityGenerator
  Set Attribute : SetAttribute  AttributeName=BatchQuantity  AttributeValue=N  EvaluatedAttributeValue={ N}
  OUT : PMIOPort  Port=1  Side=Right
  wires:
  Compare To Constant/1 -> Event-Based Entity Generator/1
  #n/1 -> Compare To Constant/1
  connections:
  Set Attribute/RConn1 -- OUT/RConn1
  Event-Based Entity Generator/RConn1 -- Set Attribute/LConn1

== system ovenLib/process control B/destroy control entity ==
  Entity Sink : EntitySink  StatNumberArrived=on
  Signal-Based Function-Call Generator : SignalBasedFunctionCallGenerator
      settings: InputPortMap=u1
  IN : PMIOPort  Port=1  Side=Left
  trigger : Outport
  wires:
  Entity Sink/1 -> Signal-Based Function-Call Generator/1
  Signal-Based Function-Call Generator/1 -> trigger/1
  connections:
  Entity Sink/LConn1 -- IN/RConn1

== system ovenLib/process control B/gate control ==
  Trigger : TriggerPort  TriggerType=function-call  VariantControl=Variant
  Function-Call Generator : simulink/Ports & Subsystems/Function-Call Generator  sample_time=-1  numberOfIterations=N
  fN : Outport
  wires:
  Function-Call Generator/1 -> fN/1

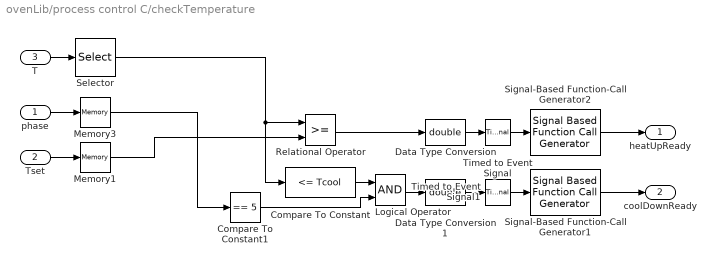
== system ovenLib/process control C/checkTemperature ==
  phase : Inport
  Tset : Inport  Port=2
  T : Inport  Port=3
  Compare To Constant : simulink/Logic and Bit Operations/Compare To Constant  relop=<=  const=Tcool  OutDataTypeStr=boolean
  Compare To Constant1 : simulink/Logic and Bit Operations/Compare To Constant  relop===  const=5  OutDataTypeStr=boolean
  Data Type Conversion : DataTypeConversion  OutDataTypeStr=double
  Data Type Conversion1 : DataTypeConversion  OutDataTypeStr=double
  Logical Operator : Logic  AllPortsSameDT=off  OutDataTypeStr=boolean
  Memory1 : Memory
  Memory3 : Memory  InheritSampleTime=on
  Relational Operator : RelationalOperator  OutDataTypeStr=boolean
  Selector : Selector  InputPortWidth=2  IndexOptions=Index vector (dialog)  Indices=[1]  OutputSizes=1
  Signal-Based Function-Call Generator1 : SignalBasedFunctionCallGenerator
      settings: InputPortMap=u1
  Signal-Based Function-Call Generator2 : SignalBasedFunctionCallGenerator
      settings: InputPortMap=u1
  Timed to Event Signal : TimedToEventSignal
  Timed to Event Signal1 : TimedToEventSignal
  heatUpReady : Outport
  coolDownReady : Outport  Port=2
  wires:
  Timed to Event Signal/1 -> Signal-Based Function-Call Generator2/1
  Signal-Based Function-Call Generator2/1 -> heatUpReady/1
  Data Type Conversion/1 -> Timed to Event Signal/1
  Relational Operator/1 -> Data Type Conversion/1
  Timed to Event Signal1/1 -> Signal-Based Function-Call Generator1/1
  Logical Operator/1 -> Data Type Conversion1/1
  Signal-Based Function-Call Generator1/1 -> coolDownReady/1
  phase/1 -> Memory3/1
  Compare To Constant/1 -> Logical Operator/1
  Compare To Constant1/1 -> Logical Operator/2
  Tset/1 -> Memory1/1
  Data Type Conversion1/1 -> Timed to Event Signal1/1
  Memory3/1 -> Compare To Constant1/1
  Memory1/1 -> Relational Operator/2
  T/1 -> Selector/1
  Selector/1 -> Compare To Constant/1, Relational Operator/1

== system ovenLib/process control C/schedTEvent ==
  newSigma : Inport
  sigma : Inport  Port=2
  Entity Departure Counter : EntityDepartureCounter
  Entity Departure Function-Call Generator1 : EntityDepartureFunctionCallGenerator
  Entity Sink2 : EntitySink
  Entity Sink3 : EntitySink
  Event-Based Entity Generator1 : EventBasedEntityGenerator  GenerateEntitiesUpon=Function call from port fcn
  Single Server1 : SingleServer  ServiceTimeFrom=Signal port t  PermitPreemption=on  SortingAttributeName=Count  SortingDirection=Descending
  wakeUp : Outport
  wires:
  Entity Departure Function-Call Generator1/1 -> wakeUp/1
  newSigma/1 -> Event-Based Entity Generator1/1
  sigma/1 -> Single Server1/1
  connections:
  Single Server1/RConn2 -- Entity Sink3/LConn1
  Entity Departure Counter/RConn1 -- Single Server1/LConn1
  Entity Departure Function-Call Generator1/RConn1 -- Entity Sink2/LConn1
  Entity Departure Counter/LConn1 -- Event-Based Entity Generator1/RConn1
  Single Server1/RConn1 -- Entity Departure Function-Call Generator1/LConn1

== system ovenLib/process physics A/phase switch ==
  phase : Inport
  Compare To Constant : simulink/Logic and Bit Operations/Compare To Constant  relop===  const=2  OutDataTypeStr=boolean
  Compare To Constant1 : simulink/Logic and Bit Operations/Compare To Constant  relop===  const=3  OutDataTypeStr=boolean
  Data Type Conversion : DataTypeConversion  OutDataTypeStr=double
  Data Type Conversion1 : DataTypeConversion  OutDataTypeStr=double
  full heating : Outport
  holding To : Outport  Port=2
  wires:
  Data Type Conversion1/1 -> holding To/1
  Compare To Constant1/1 -> Data Type Conversion1/1
  Data Type Conversion/1 -> full heating/1
  Compare To Constant/1 -> Data Type Conversion/1
  phase/1 -> Compare To Constant/1, Compare To Constant1/1

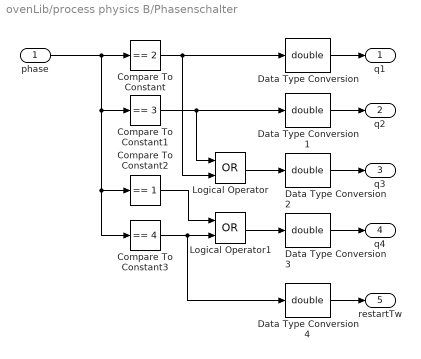
== system ovenLib/process physics B/Phasenschalter ==
  phase : Inport
  Compare To Constant : simulink/Logic and Bit Operations/Compare To Constant  relop===  const=2  OutDataTypeStr=boolean
  Compare To Constant1 : simulink/Logic and Bit Operations/Compare To Constant  relop===  const=3  OutDataTypeStr=boolean
  Compare To Constant2 : simulink/Logic and Bit Operations/Compare To Constant  relop===  const=1  OutDataTypeStr=boolean
  Compare To Constant3 : simulink/Logic and Bit Operations/Compare To Constant  relop===  const=4  OutDataTypeStr=boolean
  Data Type Conversion{,1..4} (5 alike) : DataTypeConversion  OutDataTypeStr=double
  Logical Operator : Logic  Operator=OR  AllPortsSameDT=off  OutDataTypeStr=boolean
  Logical Operator1 : Logic  Operator=OR  AllPortsSameDT=off  OutDataTypeStr=boolean
  q1 : Outport
  q2 : Outport  Port=2
  q3 : Outport  Port=3
  q4 : Outport  Port=4
  restartTw : Outport  Port=5
  wires:
  Data Type Conversion4/1 -> restartTw/1
  Compare To Constant2/1 -> Logical Operator1/1
  Compare To Constant3/1 -> Logical Operator1/2, Data Type Conversion4/1
  Logical Operator1/1 -> Data Type Conversion3/1
  Data Type Conversion3/1 -> q4/1
  Logical Operator/1 -> Data Type Conversion2/1
  Data Type Conversion2/1 -> q3/1
  Data Type Conversion1/1 -> q2/1
  Compare To Constant1/1 -> Data Type Conversion1/1, Logical Operator/1
  Data Type Conversion/1 -> q1/1
  Compare To Constant/1 -> Data Type Conversion/1, Logical Operator/2
  phase/1 -> Compare To Constant/1, Compare To Constant1/1, Compare To Constant2/1, Compare To Constant3/1

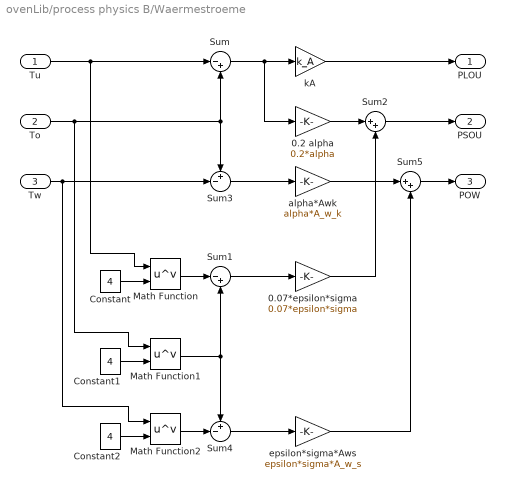
== system ovenLib/process physics B/Waermestroeme ==
  Tu : Inport
  To : Inport  Port=2
  Tw : Inport  Port=3
  0.07*epsilon*sigma : Gain  Gain=0.07*epsilon*sigma
  0.2 alpha : Gain  Gain=0.2*alpha
  Constant : Constant  Value=4
  Constant1 : Constant  Value=4
  Constant2 : Constant  Value=4
  Math Function : Math  Operator=pow  SaturateOnIntegerOverflow=on
  Math Function1 : Math  Operator=pow  SaturateOnIntegerOverflow=on
  Math Function2 : Math  Operator=pow  SaturateOnIntegerOverflow=on
  Sum : Sum  Inputs=|-+
  Sum1 : Sum  Inputs=|-+
  Sum2 : Sum  Inputs=|++
  Sum3 : Sum  Inputs=+-|
  Sum4 : Sum  Inputs=+-|
  Sum5 : Sum  Inputs=|++
  alpha*Awk : Gain  Gain=alpha*A_w_k
  epsilon*sigma*Aws : Gain  Gain=epsilon*sigma*A_w_s
  kA : Gain  Gain=k_A
  PLOU : Outport
  PSOU : Outport  Port=2
  POW : Outport  Port=3
  wires:
  Sum5/1 -> POW/1
  epsilon*sigma*Aws/1 -> Sum5/2
  alpha*Awk/1 -> Sum5/1
  Sum4/1 -> epsilon*sigma*Aws/1
  Math Function2/1 -> Sum4/2
  Sum3/1 -> alpha*Awk/1
  Sum2/1 -> PSOU/1
  0.07*epsilon*sigma/1 -> Sum2/2
  0.2 alpha/1 -> Sum2/1
  Sum1/1 -> 0.07*epsilon*sigma/1
  Math Function/1 -> Sum1/1
  Math Function1/1 -> Sum4/1, Sum1/2
  Tw/1 -> Math Function2/1, Sum3/2
  Constant2/1 -> Math Function2/2
  Constant1/1 -> Math Function1/2
  Constant/1 -> Math Function/2
  kA/1 -> PLOU/1
  Tu/1 -> Sum/1, Math Function/1
  To/1 -> Sum/2, Sum3/1, Math Function1/1
  Sum/1 -> kA/1, 0.2 alpha/1

== system ovenLib/process physics C/Fixed T ==
  Conductive Heat Transfer10 : fl_lib/Thermal/Thermal Elements/Conductive Heat Transfer  area=10 m^2  thickness=1 m  th_cond=10000 W/(m*K)  Q_specify=off  Q_priority=High  Q=0 J/s  T_specify=off  T_priority=High  T=0 K
  Ideal Temperature Source : fl_lib/Thermal/Thermal Sources/Ideal Temperature Source
  PS Constant : fl_lib/Physical Signals/Sources/PS Constant  constant=Tu + T0C
  Thermal Reference : fl_lib/Thermal/Thermal Elements/Thermal Reference
  Port : PMIOPort  Port=1  Side=Right
  connections:
  Ideal Temperature Source/LConn1 -- Conductive Heat Transfer10/RConn1
  Thermal Reference/LConn1 -- Ideal Temperature Source/RConn2
  PS Constant/RConn1 -- Ideal Temperature Source/RConn1
  Conductive Heat Transfer10/LConn1 -- Port/RConn1

== system ovenLib/process physics C/Heating Power ==
  Qzu0 : Inport
  q2 : Inport  Port=2
  P_LOU : Inport  Port=3
  P_OW : Inport  Port=4
  1/eta_o : Gain  Gain=1/etaO
  Eh : Integrator
  Gain1 : Gain  Gain=1e-3
  Gain2 : Gain  Gain=1e-3/3600
  Product : Product
  Sum2 : Sum  Inputs=|++
  Sum3 : Sum  Inputs=|++
  in Celsius1 : Bias  Bias=Pgrund
  P(t) [kW] : Outport
  E(t) [kWh] : Outport  Port=2
  wires:
  Gain2/1 -> E(t) [kWh]/1
  Eh/1 -> Gain2/1
  in Celsius1/1 -> Gain1/1, Eh/1
  Gain1/1 -> P(t) [kW]/1
  q2/1 -> Product/1
  Product/1 -> Sum3/2
  Qzu0/1 -> Sum3/1
  Sum3/1 -> 1/eta_o/1
  1/eta_o/1 -> in Celsius1/1
  P_LOU/1 -> Sum2/1
  P_OW/1 -> Sum2/2
  Sum2/1 -> Product/2

== system ovenLib/process physics C/Hold T ==
  Ideal Heat Flow Source : fl_lib/Thermal/Thermal Sources/Ideal Heat Flow Source
  PS Product : fl_lib/Physical Signals/Functions/PS Product
  Thermal Reference1 : fl_lib/Thermal/Thermal Elements/Thermal Reference
  Port : PMIOPort  Port=1  Side=Right
  Qzu : PMIOPort  Port=2  Side=Left
  control : PMIOPort  Port=3  Side=Left
  connections:
  Ideal Heat Flow Source/LConn1 -- Port/RConn1
  Qzu/RConn1 -- PS Product/LConn2
  control/RConn1 -- PS Product/LConn1
  PS Product/RConn1 -- Ideal Heat Flow Source/RConn1
  Thermal Reference1/LConn1 -- Ideal Heat Flow Source/RConn2

== system ovenLib/process physics C/Ph ==
  Ideal Heat Flow Sensor1 : fl_lib/Thermal/Thermal Sensors/Ideal Heat Flow Sensor
  Ideal Heat Flow Source : fl_lib/Thermal/Thermal Sources/Ideal Heat Flow Source
  PS-Simulink Converter : nesl_utility/PS-Simulink Converter  PhysicalDomain=network_engine_domain  SubClassName=ps_output  LeftPortType=input  RightPortType=output  PseudoPeriodic=off  Frequencies=[]  Unit=1  AffineConversion=off
  Qzu0 : fl_lib/Physical Signals/Functions/PS Gain  gain=PH*etaO
  Thermal Reference1 : fl_lib/Thermal/Thermal Elements/Thermal Reference
  Oven : PMIOPort  Port=1  Side=Right
  control : PMIOPort  Port=2  Side=Left
  tag scope: Qzu0=global
  wires:
  PS-Simulink Converter/1 -> [Qzu0]
  connections:
  PS-Simulink Converter/LConn1 -- Ideal Heat Flow Sensor1/RConn1
  Ideal Heat Flow Sensor1/RConn2 -- Oven/RConn1
  Ideal Heat Flow Source/LConn1 -- Ideal Heat Flow Sensor1/LConn1
  Thermal Reference1/LConn1 -- Ideal Heat Flow Source/RConn2
  Qzu0/RConn1 -- Ideal Heat Flow Source/RConn1
  control/RConn1 -- Qzu0/LConn1

== system ovenLib/process physics C/Set T ==
  Perfect Insulator : fl_lib/Thermal/Thermal Elements/Perfect Insulator  T_specify=off  T_priority=High  T=0 K
  Tfix : Subsystem
  ThermoSwitch : PJPhysLib_lib/ThermoSwitch  G=1e-4 W/K  Tref=300 K  Q1_specify=off  Q1_priority=High  Q1=0 J/s  Q2_specify=off  Q2_priority=High  Q2=0 J/s  Q_specify=off  Q_priority=High  Q=0 J/s
  Port : PMIOPort  Port=1  Side=Right
  control : PMIOPort  Port=2  Side=Left
  T : PMIOPort  Port=3  Side=Left
  connections:
  T/RConn1 -- Tfix/LConn1
  Tfix/RConn1 -- ThermoSwitch/LConn2
  control/RConn1 -- ThermoSwitch/LConn3
  Perfect Insulator/LConn1 -- ThermoSwitch/LConn1
  ThermoSwitch/RConn1 -- Port/RConn1

== system ovenLib/process physics C/T measurement ==
  Mux : Mux  Inputs=2
  T sensor 1 : Subsystem
  T sensor 2 : Subsystem
  to Celsius : Bias  Bias=-T0C
  Conn1 : PMIOPort  Port=1  Side=Left
  Conn2 : PMIOPort  Port=2  Side=Left
  Out1 : Outport
  wires:
  Mux/1 -> to Celsius/1
  T sensor 2/1(T) -> Mux/2
  to Celsius/1 -> Out1/1
  T sensor 1/1(T) -> Mux/1
  connections:
  T sensor 1/LConn1 -- Conn1/RConn1
  T sensor 2/LConn1 -- Conn2/RConn1

== system ovenLib/process physics C/conduction OE ==
  Conductive Heat Transfer : fl_lib/Thermal/Thermal Elements/Conductive Heat Transfer  area=1 m^2  thickness=1 m  th_cond=k_A W/(m*K)  Q_specify=off  Q_priority=High  Q=0 J/s  T_specify=off  T_priority=High  T=0 K
  Ideal Heat Flow Sensor1 : fl_lib/Thermal/Thermal Sensors/Ideal Heat Flow Sensor
  PS-Simulink Converter : nesl_utility/PS-Simulink Converter  PhysicalDomain=network_engine_domain  SubClassName=ps_output  LeftPortType=input  RightPortType=output  PseudoPeriodic=off  Frequencies=[]  Unit=1  AffineConversion=off
  Env : PMIOPort  Port=1  Side=Left
  Oven : PMIOPort  Port=2  Side=Right
  P_LOU : PMIOPort  Port=3  Side=Right
  tag scope: P_LOU=global
  wires:
  PS-Simulink Converter/1 -> [P_LOU]
  connections:
  Ideal Heat Flow Sensor1/RConn2 -- Conductive Heat Transfer/RConn1
  P_LOU/RConn1 -- PS-Simulink Converter/LConn1 -- Ideal Heat Flow Sensor1/RConn1
  Conductive Heat Transfer/LConn1 -- Env/RConn1
  Ideal Heat Flow Sensor1/LConn1 -- Oven/RConn1

== system ovenLib/process physics C/conv + rad. OL ==
  Convective Heat Transfer : fl_lib/Thermal/Thermal Elements/Convective Heat Transfer  area=A_w_k m^2  heat_tr_coeff=alpha W/(m^2 * K)  Q_specify=off  Q_priority=High  Q=0 J/s  T_specify=off  T_priority=High  T=0 K
  Ideal Heat Flow Sensor : fl_lib/Thermal/Thermal Sensors/Ideal Heat Flow Sensor
  PS-Simulink Converter : nesl_utility/PS-Simulink Converter  PhysicalDomain=network_engine_domain  SubClassName=ps_output  LeftPortType=input  RightPortType=output  PseudoPeriodic=off  Frequencies=[]  Unit=1  AffineConversion=off
  Perfect Insulator : fl_lib/Thermal/Thermal Elements/Perfect Insulator  T_specify=off  T_priority=High  T=0 K
  Radiative Heat Transfer : fl_lib/Thermal/Thermal Elements/Radiative Heat Transfer  area=A_w_s m^2  rad_tr_coeff=epsilon*sigma W/(m^2*K^4)  Q_specify=off  Q_priority=High  Q=0 J/s  T_specify=off  T_priority=High  T=0 K
  ThermoSwitch : PJPhysLib_lib/ThermoSwitch  G=1e-4 W/K  Tref=300 K  Q1_specify=off  Q1_priority=High  Q1=0 J/s  Q2_specify=off  Q2_priority=High  Q2=0 J/s  Q_specify=off  Q_priority=High  Q=0 J/s
  P_OW : PMIOPort  Port=1  Side=Right
  Oven : PMIOPort  Port=2  Side=Right
  control : PMIOPort  Port=3  Side=Left
  Load : PMIOPort  Port=4  Side=Left
  tag scope: P_OW=global
  wires:
  PS-Simulink Converter/1 -> [P_OW]
  connections:
  Ideal Heat Flow Sensor/RConn1 -- PS-Simulink Converter/LConn1 -- P_OW/RConn1
  Oven/RConn1 -- Ideal Heat Flow Sensor/LConn1
  Convective Heat Transfer/RConn1 -- ThermoSwitch/LConn2 -- Radiative Heat Transfer/RConn1
  Radiative Heat Transfer/LConn1 -- Ideal Heat Flow Sensor/RConn2 -- Convective Heat Transfer/LConn1
  control/RConn1 -- ThermoSwitch/LConn3
  Load/RConn1 -- ThermoSwitch/RConn1
  Perfect Insulator/LConn1 -- ThermoSwitch/LConn1

== system ovenLib/process physics C/conv + rad. OE ==
  Convective Heat Transfer : fl_lib/Thermal/Thermal Elements/Convective Heat Transfer  area=0.2 m^2  heat_tr_coeff=alpha W/(m^2 * K)  Q_specify=off  Q_priority=High  Q=0 J/s  T_specify=off  T_priority=High  T=0 K
  Perfect Insulator : fl_lib/Thermal/Thermal Elements/Perfect Insulator  T_specify=off  T_priority=High  T=0 K
  Radiative Heat Transfer : fl_lib/Thermal/Thermal Elements/Radiative Heat Transfer  area=0.07 m^2  rad_tr_coeff=epsilon*sigma W/(m^2*K^4)  Q_specify=off  Q_priority=High  Q=0 J/s  T_specify=off  T_priority=High  T=0 K
  ThermoSwitch : PJPhysLib_lib/ThermoSwitch  G=1e-4 W/K  Tref=300 K  Q1_specify=off  Q1_priority=High  Q1=0 J/s  Q2_specify=off  Q2_priority=High  Q2=0 J/s  Q_specify=off  Q_priority=High  Q=0 J/s
  Oven : PMIOPort  Port=1  Side=Right
  Env : PMIOPort  Port=2  Side=Left
  control : PMIOPort  Port=3  Side=Left
  connections:
  ThermoSwitch/LConn2 -- Radiative Heat Transfer/RConn1 -- Convective Heat Transfer/RConn1
  Oven/RConn1 -- Convective Heat Transfer/LConn1 -- Radiative Heat Transfer/LConn1
  control/RConn1 -- ThermoSwitch/LConn3
  Env/RConn1 -- ThermoSwitch/RConn1
  Perfect Insulator/LConn1 -- ThermoSwitch/LConn1
